simulink model "custom_mpc"  (R2019a)
settings: Solver=VariableStepAuto  StartTime=0.0  StopTime=10.0  RelTol=1e-3
libraries: mpclib x1
settings Model: Creator=colson  LastModifiedBy=colson

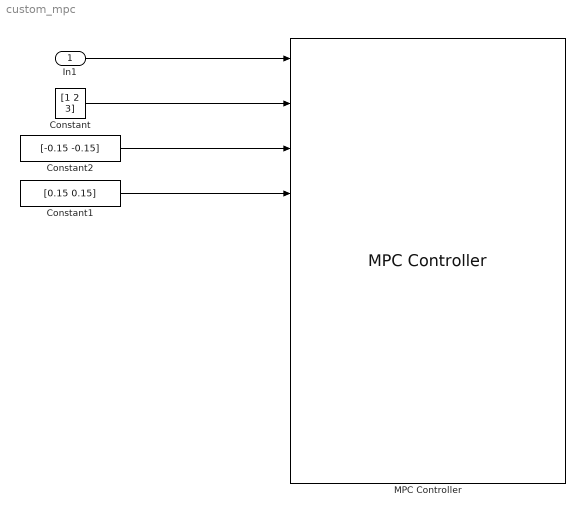
== system custom_mpc ==
  In1 : Inport
  Constant : Constant  Value=[1 2 3]
  Constant1 : Constant  Value=[0.15 0.15]
  Constant2 : Constant  Value=[-0.15 -0.15]
  MPC Controller : mpclib/MPC Controller  SCDEnableBlockLinearizationSpecification=on  is_multiple=0  enable_value=0  return_u0=off  updateMPCinCallerWorkspace=on  md_inport=off  mv_inport=off  uref_inport=on  return_cost=on  return_mvseq=on  return_qpstatus=on  return_xseq=on  return_state=on  return_ovseq=on  state_inport=off  umin_inport=on  umax_inport=on  ymin_inport=on  ymax_inport=on  cc_inport=on  ywt_inport=off  uwt_inport=off  duwt_inport=off  rhoeps_inport=off  pm_inport=off  MaximumP=10  HorizonChoice=FixedHorizon  n_ts=1  n_p=10  n_mv=1  n_md=1  n_ud=0  n_mo=1  n_uo=0  BlockDataType=double  SampleTimeInherited=off  switch_inport=off
      settings: SourceProductName=MATLAB Runtime - Model Predictive Control Toolbox Addin  SourceProductBaseCode=Missing
  wires:
  In1/1 -> MPC Controller/1
  Constant/1 -> MPC Controller/2
  Constant2/1 -> MPC Controller/3
  Constant1/1 -> MPC Controller/4
